simulink model "dynmodelinglinearmpc"  (R2019a)
settings: Solver=FixedStepAuto  StartTime=0.0  StopTime=25  RelTol=1e-3
model workspace (MAT data in the model file):
  op_trim1 : opcond.OperatingReport (value not decoded)
undefined symbols (not defined in the file or in its folder): dt, rx, ry
libraries: mpclib x1, mobileRoboticsLib x1
settings Model: Creator=Malicious  LastModifiedBy=colson
settings DataIOCC: ExternalInput=getinputstruct(op_trim1)  InitialState=getstatestruct(op_trim1)  LoadExternalInput=on  ReturnWorkspaceOutputs=off
settings DebuggingCC: PregeneratedLibrarySubsystemCodeDiagnostic=none  ArithmeticOperatorsInVariantConditions=warning
settings SFSimCC: SimUseLocalCustomCode=off
settings RTWCC: RTWUseLocalCustomCode=off

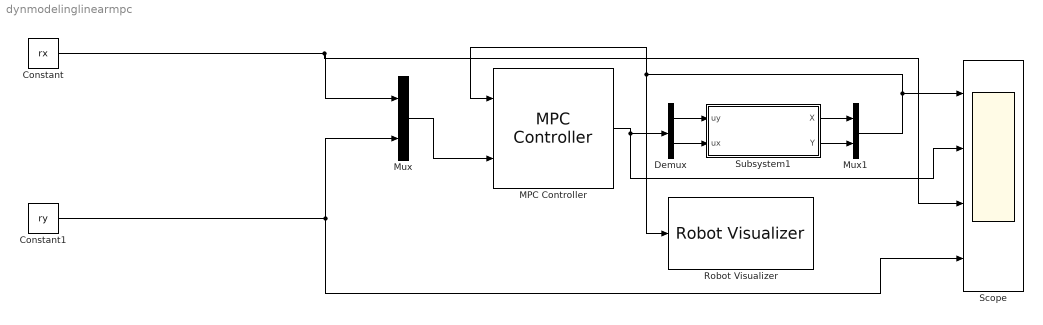
== system dynmodelinglinearmpc ==
  Constant : Constant  Value=rx
  Constant1 : Constant  Value=ry
  Demux : Demux  Outputs=2
  MPC Controller : mpclib/MPC Controller  SCDEnableBlockLinearizationSpecification=on  mpcobj=mpc1  is_multiple=0  enable_value=0  return_u0=off  updateMPCinCallerWorkspace=on  md_inport=off  mv_inport=off  uref_inport=off  return_cost=off  return_mvseq=off  return_qpstatus=off  return_xseq=off  return_state=off  return_ovseq=off  state_inport=off  umin_inport=off  umax_inport=off  ymin_inport=off  ymax_inport=off  cc_inport=off  ywt_inport=off  uwt_inport=off  duwt_inport=off  rhoeps_inport=off  pm_inport=off  MaximumP=10  HorizonChoice=FixedHorizon  n_ts=0.1  n_p=31  n_mv=2  n_md=0  n_ud=0  n_mo=2  n_uo=0  BlockDataType=double  SampleTimeInherited=off  switch_inport=off
  Mux : Mux  Inputs=2
  Mux1 : Mux  Inputs=2
  Robot Visualizer : mobileRoboticsLib/Environments/Robot Visualizer  robotRadius=0.2  showTrajectory=on  hasWaypoints=off  hasLidar=off  sensorOffset=[ 0, 0 ]  scanAngles=[ -pi/4, 0, pi/4 ]  hasObjDetector=off  objDetectorOffset=[ 0, 0 ]  objDetectorAngle=0  objDetectorFOV=pi/4  objDetectorMaxRange=5  objectColors=[ 1, 0, 0; 0, 1, 0; 0, 0, 1 ]  objectMarkers=s
      settings: SourceProductName=Mobile Robotics Simulation Library
  Scope : Scope  NumInputPorts=4
  Subsystem1 : Subsystem
  wires:
  MPC Controller/1 -> Demux/1, Scope/2
  Mux1/1 -> MPC Controller/1, Robot Visualizer/1, Scope/1
  Mux/1 -> MPC Controller/2
  Subsystem1/2(Y) -> Mux1/2
  Subsystem1/1(X) -> Mux1/1
  Demux/1 -> Subsystem1/1(uy)
  Demux/2 -> Subsystem1/2(ux)
  Constant1/1 -> Scope/4, Mux/2
  Constant/1 -> Scope/3, Mux/1

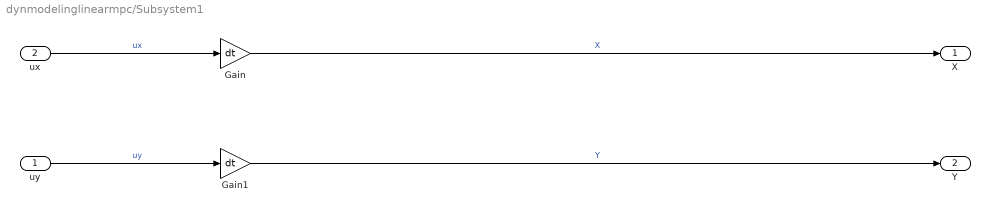
== system dynmodelinglinearmpc/Subsystem1 ==
  uy : Inport
  ux : Inport  Port=2
  Gain : Gain  Gain=dt
  Gain1 : Gain  Gain=dt
  X : Outport
  Y : Outport  Port=2
  wires:
  Gain/1 -> X/1  "X"
  Gain1/1 -> Y/1  "Y"
  ux/1 -> Gain/1  "ux"
  uy/1 -> Gain1/1  "uy"
